simulink model "siimulink"  (R2019b)
settings: Solver=VariableStepAuto  StartTime=0.0  StopTime=150  RelTol=1e-6
model workspace: external: MAT-File /home/user/Documents/Projects/MATLAB/Simulink.mat (data not in the file)
values from neighbouring files (symbols this model uses):
  J = 8.75e-05    [Model.mat]    (also in Simulink.mat; T_Funk.m)
  K_construct = 0.0175    [Model.mat]    (also in Simulink.mat)
  K_friction = 2.5e-06    [Simulink.mat]
  L = fread(fid2,Inf,'uint16','l')    [Graph_Viewer.m]    (also in Model.mat = 0.0225; Simulink.mat = 0.0225; T_Funk.m = 0.0225)
  Mtr = 0.00063125    [Model.mat]    (also in Simulink.mat; T_Funk.m)
  R = reshape(L,3, [])'    [Graph_Viewer.m]    (also in Model.mat = 16.3; Simulink.mat = 16.3)
undefined symbols (not defined in the file or in its folder): sigbuilder_block
libraries: eeGeneralControl x2
settings Model: OrderedModelArguments=off  Creator=user  LastModifiedBy=user
settings SolverCC: ConsecutiveZCsStepRelTol=10*8*eps  ZeroCrossAlgorithm=Adaptive
settings DebuggingCC: IgnoredZcDiagnostic=none

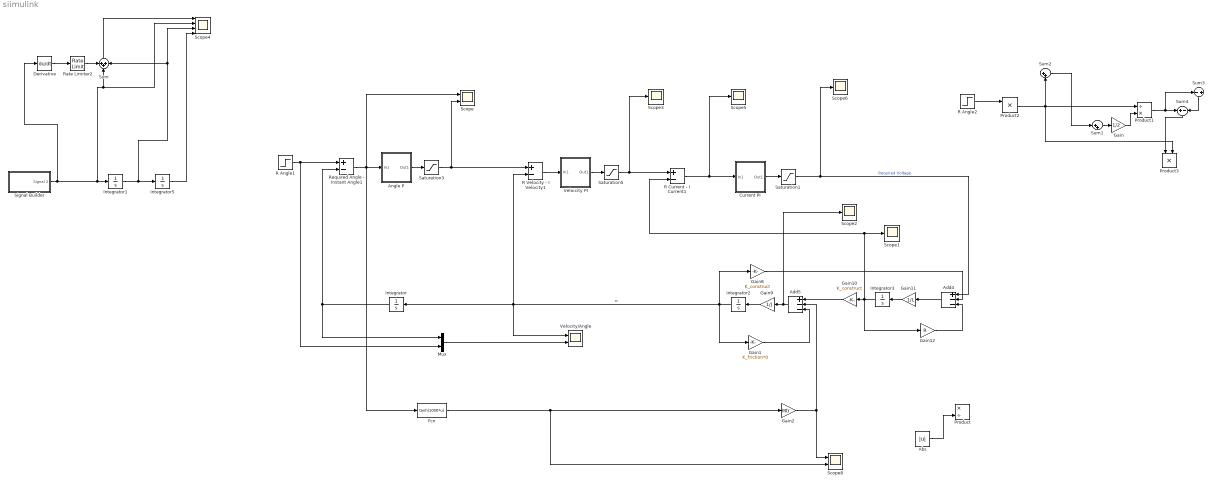
== system siimulink ==
  " Velocity/Angle" : Scope  NumInputPorts=2
  Abs : Abs
  Add4 : Sum  Inputs=+--
  Add5 : Sum  Inputs=+--
  Angle P : Subsystem
  Current PI : Subsystem
  Derivative : Derivative  CoefficientInTFapproximation=1
  Fcn : Fcn  Expr=tanh(1000*u)
  Gain : Gain  Gain=1/2
  Gain1 : Gain  Gain=K_friction*0
  Gain10 : Gain  Gain=K_construct
  Gain11 : Gain  Gain=1/L
  Gain12 : Gain  Gain=R
  Gain2 : Gain  Gain=Mtr
  Gain8 : Gain  Gain=K_construct
  Gain9 : Gain  Gain=1/J
  Integrator{,1..3,5} (5 alike) : Integrator
  Mux : Mux  Inputs=2
  Product : Product  Inputs=*/
  Product1 : Product  Inputs=/*
  Product2 : Product
  Product3 : Product
  R Angle1 : Step  Time=0  After=314.15 * 2  SampleTime=0
  R Angle2 : Step  Time=0  After=8  SampleTime=0
  R Current - I Current1 : Sum  Inputs=+-
  R Velocity - I Velocity1 : Sum  Inputs=+-
  Rate Limiter2 : RateLimiter  RisingSlewLimit=2  FallingSlewLimit=-2
  Required Angle - Instant Angle1 : Sum  Inputs=+-
  Saturation1 : Saturate  UpperLimit=12  LowerLimit=-12
  Saturation3 : Saturate  UpperLimit=100  LowerLimit=-100
  Saturation5 : Saturate  UpperLimit=1  LowerLimit=-1
  Scope : Scope  NumInputPorts=2
  Scope{1..3,5..6} (5 alike) : Scope
  Scope4 : Scope  NumInputPorts=4
  Scope8 : Scope  NumInputPorts=2
  Signal Builder : Subsystem  Tag=STV Subsys  LoadFcn=sigbuilder_block('load');  StartFcn=sigbuilder_block('start');  StopFcn=sigbuilder_block('stop');  ClipboardFcn=sigbuilder_block('clipboard');  mask(Sigbuilder block){tuvar=[0:10]}
      mask help: Simulink:masks:SigbuilderBlock_MD
      mask init:
      | if ~strcmp(get_param(bdroot(gcbh),'SimulationStatus'),'stopped') tuvar = sigbuilder_block('maskInit'); end
      settings: CopyFcn=sigbuilder_block('copy');  DeleteFcn=sigbuilder_block('delete');  ModelCloseFcn=sigbuilder_block('modelClose');  PreSaveFcn=sigbuilder_block('preSave');  PauseFcn=sigbuilder_block('pause');  ContinueFcn=sigbuilder_block('continue');  NameChangeFcn=sigbuilder_block('namechange');  OpenFcn=sigbuilder_block('open',[50.25 0 1389.75 603.75 ]);  CloseFcn=sigbuilder_block('close');
      mask Display: plot(0, 0, 100, 100,[2, 2, 32, 32, 2], [68, 8, 8, 68, 68],[32, 2], [38, 38], [32, 19, 2],[53, 60, 44], [32, 17, 17, 2],[16, 16, 31, 31]);txt = getActiveGroup(gcbh);text(2, 100, txt,'verticalAlignment', 'top');
  Sum : Sum  Inputs=+++
  Sum1 : Sum  Inputs=|++
  Sum2 : Sum  Inputs=|++
  Sum3 : Sum  Inputs=-+
  Sum4 : Sum  Inputs=+-
  Veloicity PI : Subsystem
  wires:
  Integrator2/1 -> Gain1/1, " Velocity/Angle"/1, R Velocity - I Velocity1/2, Integrator/1, Gain8/1  "w"
  Current PI/1(Out1) -> Saturation1/1
  Integrator/1 -> Mux/1, Required Angle - Instant Angle1/2
  Saturation1/1 -> Add4/1, Scope6/1  "Required Voltage"
  R Velocity - I Velocity1/1 -> Veloicity PI/1(In1)
  R Current - I Current1/1 -> Scope5/1, Current PI/1(In1)
  Angle P/1(Out1) -> Saturation3/1
  Veloicity PI/1(Out1) -> Saturation5/1
  Add4/1 -> Gain11/1
  Gain11/1 -> Integrator3/1
  Add5/1 -> Scope2/1, Gain9/1
  Gain9/1 -> Integrator2/1
  Integrator3/1 -> Scope1/1, R Current - I Current1/2, Gain12/1, Gain10/1
  Gain8/1 -> Add4/2
  Gain12/1 -> Add4/3
  Mux/1 -> " Velocity/Angle"/2
  Signal Builder/1(Signal 2) -> Derivative/1, Integrator1/1, Scope4/2, Sum/2
  Integrator1/1 -> Scope4/3, Sum/3, Integrator5/1
  Derivative/1 -> Rate Limiter2/1
  Rate Limiter2/1 -> Sum/1
  Sum/1 -> Scope4/1
  Integrator5/1 -> Scope4/4
  Saturation3/1 -> Scope/2, R Velocity - I Velocity1/1
  R Angle1/1 -> Mux/2, Required Angle - Instant Angle1/1
  Gain10/1 -> Add5/1
  Required Angle - Instant Angle1/1 -> Fcn/1, Angle P/1(In1), Scope/1
  Saturation5/1 -> Scope3/1, R Current - I Current1/1
  Gain1/1 -> Add5/3
  Gain2/1 -> Scope8/1, Add5/2
  Abs/1 -> Product/2
  Sum1/1 -> Gain/1
  Gain/1 -> Product1/2
  R Angle2/1 -> Product2/1
  Sum2/1 -> Sum1/1
  Product2/1 -> Product3/2, Product1/1, Sum2/2
  Fcn/1 -> Scope8/2, Gain2/1
  Product1/1 -> Sum4/1, Sum3/1
  Sum3/1 -> Sum4/2
  Sum4/1 -> Product3/1

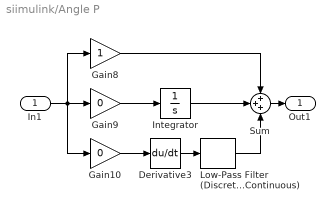
== system siimulink/Angle P ==
  In1 : Inport
  Derivative3 : Derivative
  Gain10 : Gain  Gain=0
  Gain8 : Gain
  Gain9 : Gain  Gain=0
  Integrator : Integrator  LimitOutput=on  UpperSaturationLimit=2000  LowerSaturationLimit=-2000
  Low-Pass Filter (Discrete or Continuous) : eeGeneralControl/Low-Pass Filter (Discrete or Continuous)  K=1  T=1  B=inf  A=-inf  Ts=0
      settings: SourceProductName=Simscape Electrical
  Sum : Sum  Inputs=3
  Out1 : Outport
  wires:
  Gain8/1 -> Sum/1
  Derivative3/1 -> Low-Pass Filter (Discrete or Continuous)/1
  In1/1 -> Gain9/1, Gain10/1, Gain8/1
  Gain9/1 -> Integrator/1
  Low-Pass Filter (Discrete or Continuous)/1 -> Sum/3
  Gain10/1 -> Derivative3/1
  Sum/1 -> Out1/1
  Integrator/1 -> Sum/2

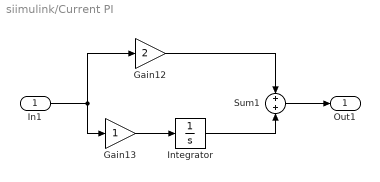
== system siimulink/Current PI ==
  In1 : Inport
  Gain12 : Gain  Gain=2
  Gain13 : Gain
  Integrator : Integrator  LimitOutput=on  UpperSaturationLimit=12  LowerSaturationLimit=-12
  Sum1 : Sum  Inputs=2
  Out1 : Outport
  wires:
  In1/1 -> Gain13/1, Gain12/1
  Gain13/1 -> Integrator/1
  Gain12/1 -> Sum1/1
  Sum1/1 -> Out1/1
  Integrator/1 -> Sum1/2

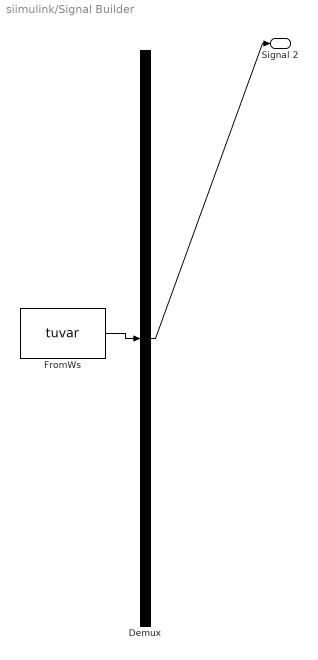
== system siimulink/Signal Builder ==
  Demux : Demux  Tag=STV Demux  Outputs=1
  FromWs : FromWorkspace  Tag=STV FromWs  VariableName=tuvar  SampleTime=0
      SigBuilderData=|
      | common.afterFinalStr = 'Extrapolate'
      | common.sampleTime = 0
      | dataSet.timeRange = [0 10]
      | dataSet.name = 'Group 1'
      | sbobj.Groups.Name = 'Group 1'
      | sbobj.Groups.Signals.Name = 'Signal 2'
      | sbobj.Groups.Signals.XData = [0 1 1 3 3 4 4 6 6 10]
      | sbobj.Groups.Signals.YData = [0 0 10 10 0 0 -10 -10 0 0]
  Signal 2 : Outport  Tag=STV Outport
  wires:
  FromWs/1 -> Demux/1
  Demux/1 -> Signal 2/1

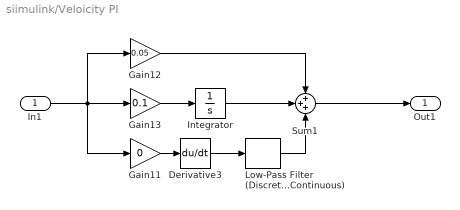
== system siimulink/Veloicity PI ==
  In1 : Inport
  Derivative3 : Derivative
  Gain11 : Gain  Gain=0
  Gain12 : Gain  Gain=0.05
  Gain13 : Gain  Gain=0.1
  Integrator : Integrator  LimitOutput=on  UpperSaturationLimit=1  LowerSaturationLimit=-1
  Low-Pass Filter (Discrete or Continuous) : eeGeneralControl/Low-Pass Filter (Discrete or Continuous)  K=1  T=1  B=inf  A=-inf  Ts=0
      settings: SourceProductName=Simscape Electrical
  Sum1 : Sum  Inputs=3
  Out1 : Outport
  wires:
  Low-Pass Filter (Discrete or Continuous)/1 -> Sum1/3
  Derivative3/1 -> Low-Pass Filter (Discrete or Continuous)/1
  In1/1 -> Gain13/1, Gain11/1, Gain12/1
  Gain13/1 -> Integrator/1
  Gain12/1 -> Sum1/1
  Gain11/1 -> Derivative3/1
  Sum1/1 -> Out1/1
  Integrator/1 -> Sum1/2
